simulink model "ctrlauto_tp1_o"  (R2019b)
settings: Solver=ode45  StartTime=0.0  StopTime=6  FixedStep=0.001  RelTol=1e-3
undefined symbols (not defined in the file or in its folder): A, B, C, D, Ts, ueq, xeq, yref
settings Model: Creator=aghersin  LastModifiedBy=rochi
settings DataIOCC: ReturnWorkspaceOutputs=off
settings DebuggingCC: ArithmeticOperatorsInVariantConditions=warning
settings SFSimCC: SimUseLocalCustomCode=off  CustomCodeUndefinedFunction=UseInterfaceOnly
settings RTWCC: RTWUseLocalCustomCode=off

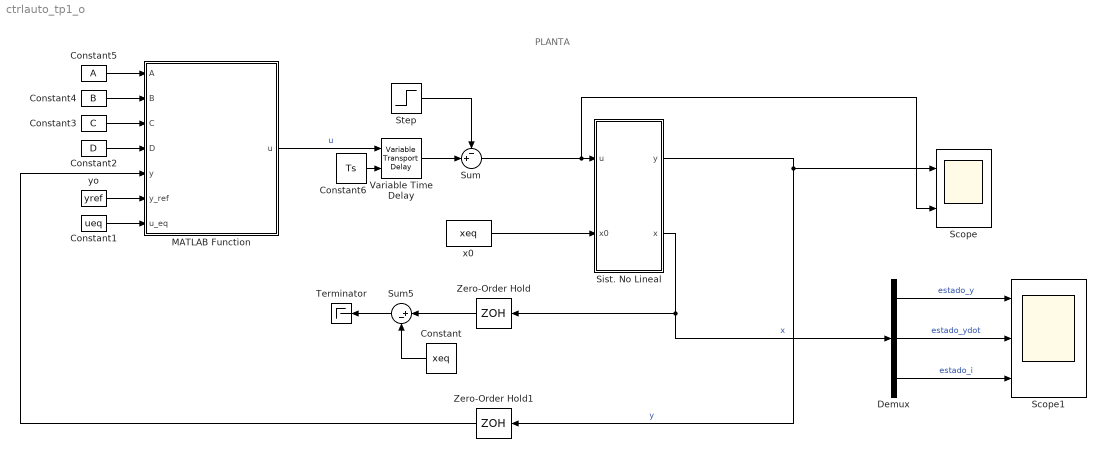
== system ctrlauto_tp1_o ==
  note: PLANTA
  Constant : Constant  Value=xeq
  Constant1 : Constant  Value=ueq
  Constant2 : Constant  Value=D
  Constant3 : Constant  Value=C
  Constant4 : Constant  Value=B
  Constant5 : Constant  Value=A
  Constant6 : Constant  Value=Ts
  Demux : Demux  Outputs=3
  MATLAB Function : MATLAB Function  TreatAsAtomicUnit=on
  Scope : Scope  NumInputPorts=2
  Scope1 : Scope  NumInputPorts=3
  "Sist. No Lineal " : Subsystem
  Step : Step  Time=3  After=0.1  SampleTime=0
  Sum : Sum  Inputs=-+|
  Sum5 : Sum  Inputs=|+-
  Terminator : Terminator
  Variable Time Delay : VariableTransportDelay
  Zero-Order Hold : ZeroOrderHold  SampleTime=Ts
  Zero-Order Hold1 : ZeroOrderHold  SampleTime=Ts
  x0 : Constant  Value=xeq
  yo : Constant  Value=yref
  wires:
  "Sist. No Lineal "/2(x) -> Demux/1, Zero-Order Hold/1  "x"
  "Sist. No Lineal "/1(y) -> Zero-Order Hold1/1, Scope/1  "y"
  x0/1 -> "Sist. No Lineal "/2(x0)
  Constant/1 -> Sum5/2
  Demux/3 -> Scope1/3  "estado_i"
  Demux/2 -> Scope1/2  "estado_ydot"
  Demux/1 -> Scope1/1  "estado_y"
  Step/1 -> Sum/1
  Sum/1 -> Scope/2, "Sist. No Lineal "/1(u)
  Zero-Order Hold/1 -> Sum5/1
  Sum5/1 -> Terminator/1
  yo/1 -> MATLAB Function/6(y_ref)
  Constant1/1 -> MATLAB Function/7(u_eq)
  Constant2/1 -> MATLAB Function/4(D)
  Constant3/1 -> MATLAB Function/3(C)
  Constant4/1 -> MATLAB Function/2(B)
  Constant5/1 -> MATLAB Function/1(A)
  Zero-Order Hold1/1 -> MATLAB Function/5(y)
  MATLAB Function/1(u) -> Variable Time Delay/1  "u"
  Constant6/1 -> Variable Time Delay/2
  Variable Time Delay/1 -> Sum/2

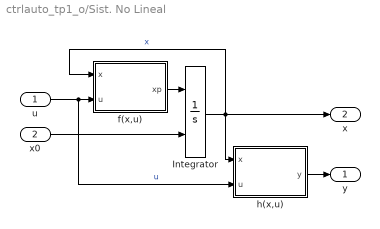
== system ctrlauto_tp1_o/Sist. No Lineal  ==
  u : Inport
  x0 : Inport  Port=2
  Integrator : Integrator  InitialConditionSource=external  ZeroCross=off
  f(x,u) : MATLAB Function  TreatAsAtomicUnit=on
  h(x,u) : MATLAB Function  TreatAsAtomicUnit=on
  y : Outport  VectorParamsAs1DForOutWhenUnconnected=off
  x : Outport  Port=2  VectorParamsAs1DForOutWhenUnconnected=off
  wires:
  h(x,u)/1(y) -> y/1
  u/1 -> h(x,u)/2(u), f(x,u)/2(u)  "u"
  f(x,u)/1(xp) -> Integrator/1
  Integrator/1 -> h(x,u)/1(x), x/1, f(x,u)/1(x)  "x"
  x0/1 -> Integrator/2

== matlab function ctrlauto_tp1_o/Sist. No Lineal /f(x,u) ==
  data: x input; u input; xp output
function xp = f(x,u)

xp1 = x(2);
xp2 = (5*(x(3) + 2)^2)/(2*(x(1) - 1)^2) ...
    - (5*(x(3) - 2)^2)/(2*(x(1) + 1)^2) - 10; 
xp3 = - 4*x(3)^2 + u;

xp = [xp1; xp2; xp3];

== matlab function ctrlauto_tp1_o/Sist. No Lineal /h(x,u) ==
  data: x input; u input; y output
function y = h(x,u)

y=x(1);

== matlab function ctrlauto_tp1_o/MATLAB Function ==
  data: A input; u output; B input; C input; D input; y input; y_ref input; u_eq input
function u = fcn(A, B, C, D, y, y_ref, u_eq)

persistent x_dot;
if isempty(x_dot)
    x_dot = [0;0;0;0];
end

error = -(y-y_ref);
u = transpose(C)*x_dot+D*error + u_eq;
x_dot = A*x_dot+B*error;

end
